simulink model "Worked_Example_10_3"  (R2024b)
settings: Solver=VariableStepAuto  StartTime=0.0  StopTime=12  RelTol=1e-3
settings Model: Creator=GH-X-ST  LastModifiedBy=GH-X-ST

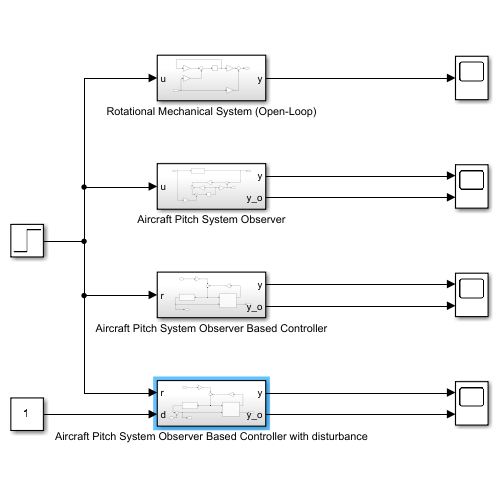
[thumbnail: Simulink's stored preview of the top-level diagram]
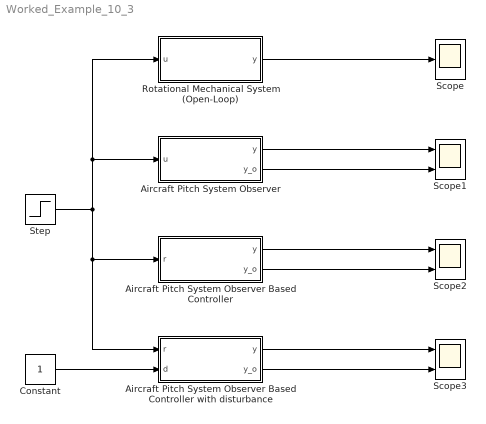
== system Worked_Example_10_3 ==
  Aircraft Pitch System Observer : Subsystem
  Aircraft Pitch System Observer Based Controller : Subsystem
  Aircraft Pitch System Observer Based Controller with disturbance : Subsystem
  Constant : Constant
  Rotational Mechanical System (Open-Loop) : Subsystem
  Scope : Scope
  Scope1 : Scope  NumInputPorts=2
  Scope2 : Scope  NumInputPorts=2
  Scope3 : Scope  NumInputPorts=2
  Step : Step  SampleTime=0
  wires:
  Step/1 -> Rotational Mechanical System (Open-Loop)/1(u), Aircraft Pitch System Observer/1(u), Aircraft Pitch System Observer Based Controller with disturbance/1(r), Aircraft Pitch System Observer Based Controller/1(r)
  Rotational Mechanical System (Open-Loop)/1(y) -> Scope/1
  Aircraft Pitch System Observer/1(y) -> Scope1/1
  Aircraft Pitch System Observer/2(y_o) -> Scope1/2
  Aircraft Pitch System Observer Based Controller/1(y) -> Scope2/1
  Aircraft Pitch System Observer Based Controller/2(y_o) -> Scope2/2
  Constant/1 -> Aircraft Pitch System Observer Based Controller with disturbance/2(d)
  Aircraft Pitch System Observer Based Controller with disturbance/1(y) -> Scope3/1
  Aircraft Pitch System Observer Based Controller with disturbance/2(y_o) -> Scope3/2

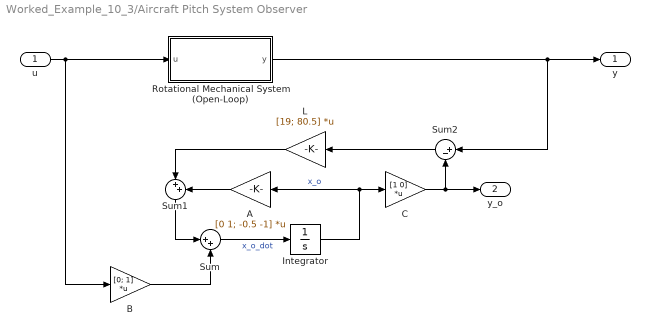
== system Worked_Example_10_3/Aircraft Pitch System Observer ==
  u : Inport
  A : Gain  Gain=[0 1; -0.5 -1]  Multiplication=Matrix(K*u)
  B : Gain  Gain=[0; 1]  Multiplication=Matrix(K*u)
  C : Gain  Gain=[1 0]  Multiplication=Matrix(K*u)
  Integrator : Integrator  InitialCondition=[0;0]
  L : Gain  Gain=[19; 80.5]  Multiplication=Matrix(K*u)
  Rotational Mechanical System (Open-Loop) : Subsystem
  Sum : Sum  Inputs=|++
  Sum1 : Sum  Inputs=|++
  Sum2 : Sum  Inputs=|+-
  y : Outport
  y_o : Outport  Port=2
  wires:
  u/1 -> Rotational Mechanical System (Open-Loop)/1(u), B/1
  Rotational Mechanical System (Open-Loop)/1(y) -> Sum2/1, y/1
  Sum/1 -> Integrator/1  "x_o_dot"
  Integrator/1 -> A/1, C/1  "x_o"
  B/1 -> Sum/2
  Sum1/1 -> Sum/1
  L/1 -> Sum1/1
  A/1 -> Sum1/2
  C/1 -> Sum2/2, y_o/1
  Sum2/1 -> L/1

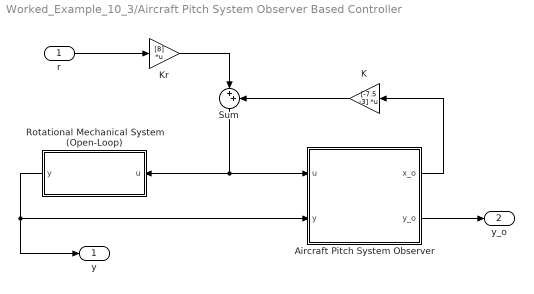
== system Worked_Example_10_3/Aircraft Pitch System Observer Based Controller ==
  r : Inport
  Aircraft Pitch System Observer : Subsystem
  K : Gain  Gain=[-7.5 -3]  Multiplication=Matrix(K*u)
  Kr : Gain  Gain=[8]  Multiplication=Matrix(K*u)
  Rotational Mechanical System (Open-Loop) : Subsystem
  Sum : Sum  Inputs=|++
  y : Outport
  y_o : Outport  Port=2
  wires:
  Aircraft Pitch System Observer/2(y_o) -> y_o/1
  Sum/1 -> Aircraft Pitch System Observer/1(u), Rotational Mechanical System (Open-Loop)/1(u)
  r/1 -> Kr/1
  Kr/1 -> Sum/1
  Rotational Mechanical System (Open-Loop)/1(y) -> y/1, Aircraft Pitch System Observer/2(y)
  Aircraft Pitch System Observer/1(x_o) -> K/1
  K/1 -> Sum/2

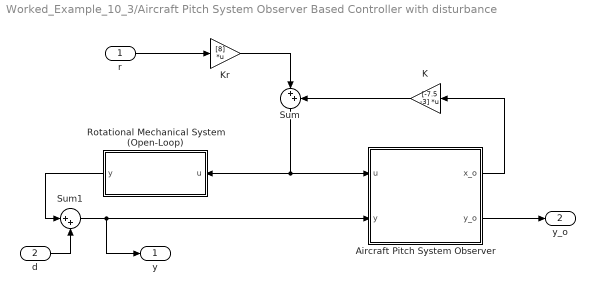
== system Worked_Example_10_3/Aircraft Pitch System Observer Based Controller with disturbance ==
  r : Inport
  d : Inport  Port=2
  Aircraft Pitch System Observer : Subsystem
  K : Gain  Gain=[-7.5 -3]  Multiplication=Matrix(K*u)
  Kr : Gain  Gain=[8]  Multiplication=Matrix(K*u)
  Rotational Mechanical System (Open-Loop) : Subsystem
  Sum : Sum  Inputs=|++
  Sum1 : Sum  Inputs=|++
  y : Outport
  y_o : Outport  Port=2
  wires:
  Aircraft Pitch System Observer/2(y_o) -> y_o/1
  Sum/1 -> Aircraft Pitch System Observer/1(u), Rotational Mechanical System (Open-Loop)/1(u)
  r/1 -> Kr/1
  Kr/1 -> Sum/1
  Aircraft Pitch System Observer/1(x_o) -> K/1
  K/1 -> Sum/2
  Rotational Mechanical System (Open-Loop)/1(y) -> Sum1/1
  Sum1/1 -> y/1, Aircraft Pitch System Observer/2(y)
  d/1 -> Sum1/2

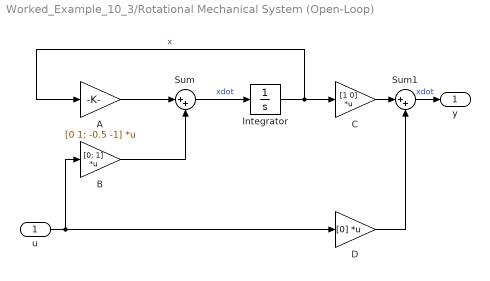
== system Worked_Example_10_3/Rotational Mechanical System (Open-Loop) ==
  u : Inport
  A : Gain  Gain=[0 1; -0.5 -1]  Multiplication=Matrix(K*u)
  B : Gain  Gain=[0; 1]  Multiplication=Matrix(K*u)
  C : Gain  Gain=[1 0]  Multiplication=Matrix(K*u)
  D : Gain  Gain=[0]  Multiplication=Matrix(K*u)
  Integrator : Integrator  InitialCondition=[1; 1]
  Sum : Sum  Inputs=|++
  Sum1 : Sum  Inputs=|++
  y : Outport
  wires:
  u/1 -> D/1, B/1
  A/1 -> Sum/1
  B/1 -> Sum/2
  Sum/1 -> Integrator/1  "xdot"
  Integrator/1 -> C/1, A/1  "x"
  C/1 -> Sum1/1
  Sum1/1 -> y/1  "xdot"
  D/1 -> Sum1/2

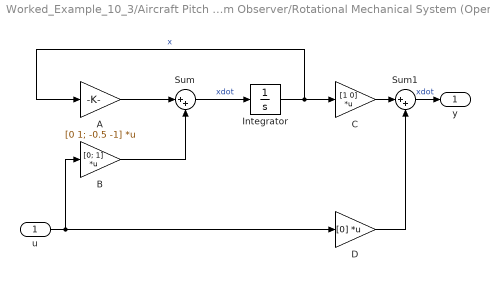
== system Worked_Example_10_3/Aircraft Pitch System Observer/Rotational Mechanical System (Open-Loop) ==
  u : Inport
  A : Gain  Gain=[0 1; -0.5 -1]  Multiplication=Matrix(K*u)
  B : Gain  Gain=[0; 1]  Multiplication=Matrix(K*u)
  C : Gain  Gain=[1 0]  Multiplication=Matrix(K*u)
  D : Gain  Gain=[0]  Multiplication=Matrix(K*u)
  Integrator : Integrator  InitialCondition=[1; 1]
  Sum : Sum  Inputs=|++
  Sum1 : Sum  Inputs=|++
  y : Outport
  wires:
  u/1 -> D/1, B/1
  A/1 -> Sum/1
  B/1 -> Sum/2
  Sum/1 -> Integrator/1  "xdot"
  Integrator/1 -> C/1, A/1  "x"
  C/1 -> Sum1/1
  Sum1/1 -> y/1  "xdot"
  D/1 -> Sum1/2

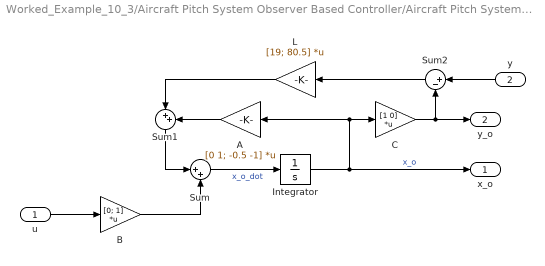
== system Worked_Example_10_3/Aircraft Pitch System Observer Based Controller/Aircraft Pitch System Observer ==
  u : Inport
  y : Inport  Port=2
  A : Gain  Gain=[0 1; -0.5 -1]  Multiplication=Matrix(K*u)
  B : Gain  Gain=[0; 1]  Multiplication=Matrix(K*u)
  C : Gain  Gain=[1 0]  Multiplication=Matrix(K*u)
  Integrator : Integrator  InitialCondition=[0;0]
  L : Gain  Gain=[19; 80.5]  Multiplication=Matrix(K*u)
  Sum : Sum  Inputs=|++
  Sum1 : Sum  Inputs=|++
  Sum2 : Sum  Inputs=|+-
  x_o : Outport
  y_o : Outport  Port=2
  wires:
  u/1 -> B/1
  y/1 -> Sum2/1
  Sum/1 -> Integrator/1  "x_o_dot"
  Integrator/1 -> x_o/1, A/1, C/1  "x_o"
  B/1 -> Sum/2
  Sum1/1 -> Sum/1
  L/1 -> Sum1/1
  A/1 -> Sum1/2
  C/1 -> Sum2/2, y_o/1
  Sum2/1 -> L/1

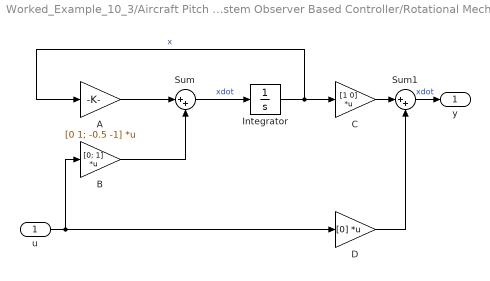
== system Worked_Example_10_3/Aircraft Pitch System Observer Based Controller/Rotational Mechanical System (Open-Loop) ==
  u : Inport
  A : Gain  Gain=[0 1; -0.5 -1]  Multiplication=Matrix(K*u)
  B : Gain  Gain=[0; 1]  Multiplication=Matrix(K*u)
  C : Gain  Gain=[1 0]  Multiplication=Matrix(K*u)
  D : Gain  Gain=[0]  Multiplication=Matrix(K*u)
  Integrator : Integrator  InitialCondition=[1; 1]
  Sum : Sum  Inputs=|++
  Sum1 : Sum  Inputs=|++
  y : Outport
  wires:
  u/1 -> D/1, B/1
  A/1 -> Sum/1
  B/1 -> Sum/2
  Sum/1 -> Integrator/1  "xdot"
  Integrator/1 -> C/1, A/1  "x"
  C/1 -> Sum1/1
  Sum1/1 -> y/1  "xdot"
  D/1 -> Sum1/2

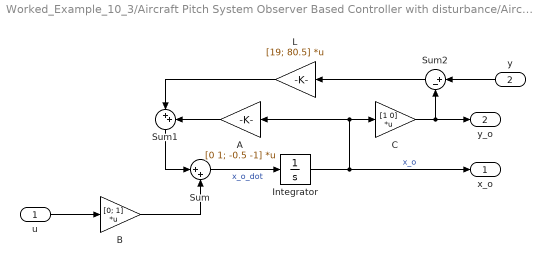
== system Worked_Example_10_3/Aircraft Pitch System Observer Based Controller with disturbance/Aircraft Pitch System Observer ==
  u : Inport
  y : Inport  Port=2
  A : Gain  Gain=[0 1; -0.5 -1]  Multiplication=Matrix(K*u)
  B : Gain  Gain=[0; 1]  Multiplication=Matrix(K*u)
  C : Gain  Gain=[1 0]  Multiplication=Matrix(K*u)
  Integrator : Integrator  InitialCondition=[0;0]
  L : Gain  Gain=[19; 80.5]  Multiplication=Matrix(K*u)
  Sum : Sum  Inputs=|++
  Sum1 : Sum  Inputs=|++
  Sum2 : Sum  Inputs=|+-
  x_o : Outport
  y_o : Outport  Port=2
  wires:
  u/1 -> B/1
  y/1 -> Sum2/1
  Sum/1 -> Integrator/1  "x_o_dot"
  Integrator/1 -> x_o/1, A/1, C/1  "x_o"
  B/1 -> Sum/2
  Sum1/1 -> Sum/1
  L/1 -> Sum1/1
  A/1 -> Sum1/2
  C/1 -> Sum2/2, y_o/1
  Sum2/1 -> L/1

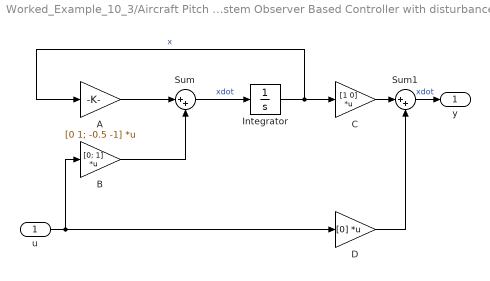
== system Worked_Example_10_3/Aircraft Pitch System Observer Based Controller with disturbance/Rotational Mechanical System (Open-Loop) ==
  u : Inport
  A : Gain  Gain=[0 1; -0.5 -1]  Multiplication=Matrix(K*u)
  B : Gain  Gain=[0; 1]  Multiplication=Matrix(K*u)
  C : Gain  Gain=[1 0]  Multiplication=Matrix(K*u)
  D : Gain  Gain=[0]  Multiplication=Matrix(K*u)
  Integrator : Integrator  InitialCondition=[1; 1]
  Sum : Sum  Inputs=|++
  Sum1 : Sum  Inputs=|++
  y : Outport
  wires:
  u/1 -> D/1, B/1
  A/1 -> Sum/1
  B/1 -> Sum/2
  Sum/1 -> Integrator/1  "xdot"
  Integrator/1 -> C/1, A/1  "x"
  C/1 -> Sum1/1
  Sum1/1 -> y/1  "xdot"
  D/1 -> Sum1/2
